simulink model "otter_traj_test"  (R2024a)
settings: Solver=FixedStepAuto  StartTime=0.0  StopTime=10.0  FixedStep=0.05  RelTol=1e-3
PostLoadFcn:
  | on_model_load
StartFcn:
  | on_model_start
StopFcn:
  | on_simulation_done
undefined symbols (not defined in the file or in its folder): ActiveScenario
libraries: csbenchlab_dist x4, mss_wrappers x3, csbenchlab_Controllers x2, ctl x1, csbenchlab_est x1, SignalEditorBlockLib x1
PostSaveFcn:
  | on_model_save
settings Model: Creator=luka  LastModifiedBy=luka

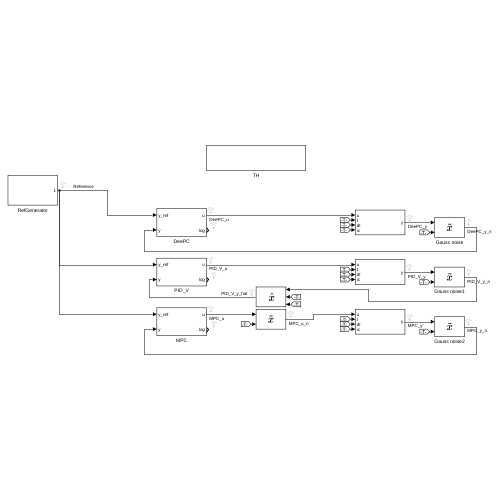
[thumbnail: Simulink's stored preview of the top-level diagram]
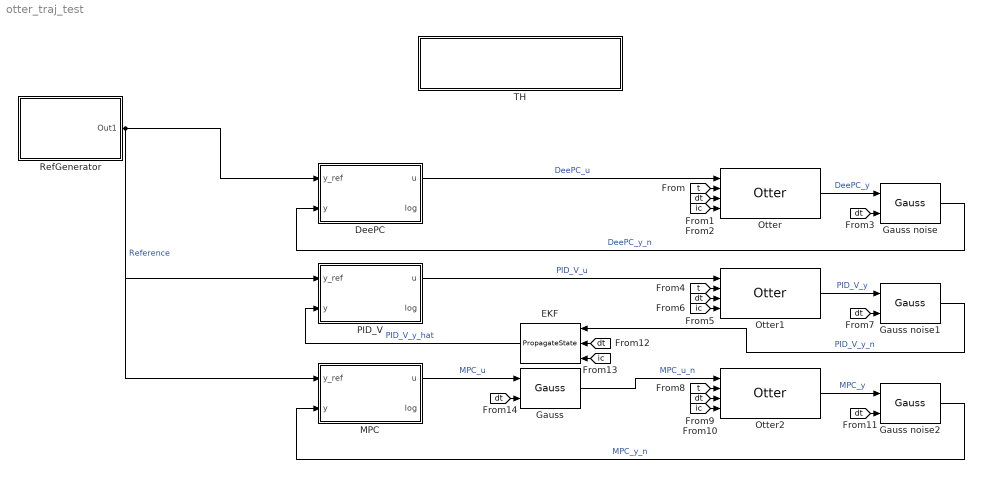
== system otter_traj_test ==
  DeePC : Subsystem
  EKF : csbenchlab_est/PropagateState  Tag=__cs_m_est;  params=PropagateState_params  data=PropagateState_data  ParamsType=PropagateState_PT  DataType=PropagateState_DT  iid__=[0]  pid__=[80 114 111 112 97 103 97 116 101 83 116 97 116 101 58 99 115 98 101 110 99 104 108 97 98]
  Gauss : csbenchlab_dist/Gauss  Tag=__cs_m_dist;  params=Gauss_params  data=Gauss_data  ParamsType=Gauss_PT  DataType=Gauss_DT  iid__=[0]  pid__=[71 97 117 115 115 58 99 115 98 101 110 99 104 108 97 98]
  Gauss noise : csbenchlab_dist/Gauss  Tag=__cs_m_dist;  params=Gauss_params  data=Gauss_data  ParamsType=Gauss_PT  DataType=Gauss_DT  iid__=[0]  pid__=[71 97 117 115 115 58 99 115 98 101 110 99 104 108 97 98]
  Gauss noise1 : csbenchlab_dist/Gauss  Tag=__cs_m_dist;  params=Gauss_params  data=Gauss_data  ParamsType=Gauss_PT  DataType=Gauss_DT  iid__=[0]  pid__=[71 97 117 115 115 58 99 115 98 101 110 99 104 108 97 98]
  Gauss noise2 : csbenchlab_dist/Gauss  Tag=__cs_m_dist;  params=Gauss_params  data=Gauss_data  ParamsType=Gauss_PT  DataType=Gauss_DT  iid__=[0]  pid__=[71 97 117 115 115 58 99 115 98 101 110 99 104 108 97 98]
  MPC : Subsystem
  Otter : mss_wrappers/Otter  Tag=system;__cs_slx_sys;  params=Otter_params_bkp  merged_params=ActiveScenario.Params
  Otter1 : mss_wrappers/Otter  Tag=system;__cs_slx_sys;  params=Otter_params_bkp  merged_params=ActiveScenario.Params
  Otter2 : mss_wrappers/Otter  Tag=system;__cs_slx_sys;  params=Otter_params_bkp  merged_params=ActiveScenario.Params
  PID_V : Subsystem
  RefGenerator : Subsystem  mask{scenario=P1}
      settings: OpenFcn=on_reference_generator_open();
      mask TypeOptions scenario: P1
      mask Callback scenario: on_reference_select;
      mask DialogControl edit_refs_btn Prompt: Edit references
      mask DialogControl edit_refs_btn Callback: on_edit_references_btn;
  TH : Subsystem
      mask DialogControl ParameterGroupVar Prompt: Params
  wires:
  [t] -> Otter/2
  [dt] -> Otter/3
  [ic] -> Otter/4
  [dt] -> Gauss noise/2
  [t] -> Otter1/2
  [dt] -> Otter1/3
  [ic] -> Otter1/4
  [dt] -> Gauss noise1/2
  [t] -> Otter2/2
  [dt] -> Otter2/3
  [ic] -> Otter2/4
  [dt] -> Gauss noise2/2
  [dt] -> EKF/2
  [ic] -> EKF/3
  [dt] -> Gauss/2
  DeePC/1(u) -> Otter/1  "DeePC_u"
  Otter/1 -> Gauss noise/1  "DeePC_y"
  Gauss noise/1 -> DeePC/2(y)  "DeePC_y_n"
  RefGenerator/1(Out1) -> DeePC/1(y_ref), PID_V/1(y_ref), MPC/1(y_ref)  "Reference"
  PID_V/1(u) -> Otter1/1  "PID_V_u"
  Otter1/1 -> Gauss noise1/1  "PID_V_y"
  Gauss noise1/1 -> EKF/1  "PID_V_y_n"
  EKF/1 -> PID_V/2(y)  "PID_V_y_hat"
  MPC/1(u) -> Gauss/1  "MPC_u"
  Gauss/1 -> Otter2/1  "MPC_u_n"
  Otter2/1 -> Gauss noise2/1  "MPC_y"
  Gauss noise2/1 -> MPC/2(y)  "MPC_y_n"

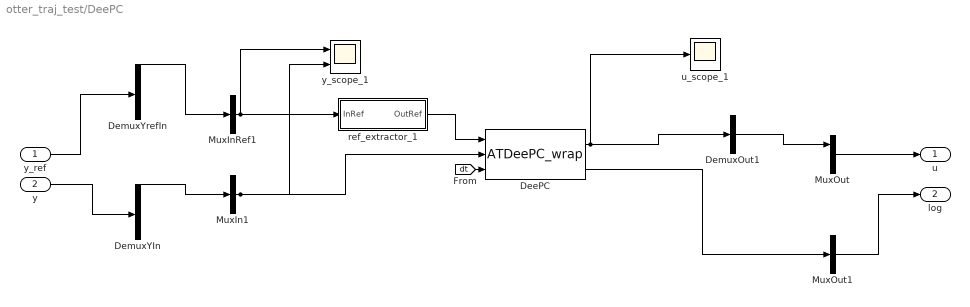
== system otter_traj_test/DeePC ==
  y_ref : Inport  PortDimensions=12
  y : Inport  Port=2  PortDimensions=12
  DeePC : ctl/ATDeePC_wrap  Tag=controller;__cs_slx_ctl;  params=ATDeePC_params  trajectory_T=0  data=0  db_params=0
  DemuxOut1 : Demux  Outputs=1
  DemuxYIn : Demux  Outputs=12
  DemuxYrefIn : Demux  Outputs=12
  MuxIn1 : Mux  Inputs=1
  MuxInRef1 : Mux  Inputs=1
  MuxOut : Mux  Inputs=2
  MuxOut1 : BusCreator  Inputs=1
  ref_extractor_1 : Subsystem
  u_scope_1 : Scope
  y_scope_1 : Scope  NumInputPorts=2
  u : Outport  PortDimensions=2
  log : Outport  Port=2
  wires:
  [dt] -> DeePC/3
  y/1 -> DemuxYIn/1
  y_ref/1 -> DemuxYrefIn/1
  MuxOut/1 -> u/1
  MuxOut1/1 -> log/1
  MuxInRef1/1 -> ref_extractor_1/1(InRef), y_scope_1/1
  ref_extractor_1/1(OutRef) -> DeePC/1
  MuxIn1/1 -> DeePC/2, y_scope_1/2
  DeePC/1 -> DemuxOut1/1, u_scope_1/1
  DeePC/2 -> MuxOut1/1
  DemuxYIn/1 -> MuxIn1/1
  DemuxYrefIn/1 -> MuxInRef1/1
  DemuxOut1/1 -> MuxOut/1

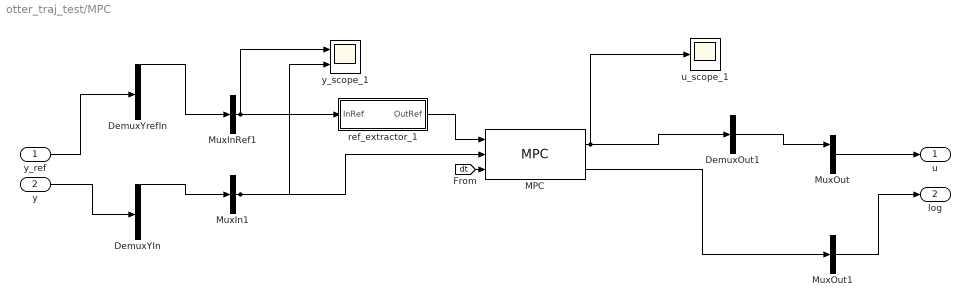
== system otter_traj_test/MPC ==
  y_ref : Inport  PortDimensions=12
  y : Inport  Port=2  PortDimensions=12
  DemuxOut1 : Demux  Outputs=1
  DemuxYIn : Demux  Outputs=12
  DemuxYrefIn : Demux  Outputs=12
  MPC : csbenchlab_Controllers/MPC  Tag=__cs_slx_ctl;  params=MPC_params
  MuxIn1 : Mux  Inputs=1
  MuxInRef1 : Mux  Inputs=1
  MuxOut : Mux  Inputs=2
  MuxOut1 : BusCreator  Inputs=1
  ref_extractor_1 : Subsystem
  u_scope_1 : Scope
  y_scope_1 : Scope  NumInputPorts=2
  u : Outport  PortDimensions=2
  log : Outport  Port=2
  wires:
  [dt] -> MPC/3
  y/1 -> DemuxYIn/1
  y_ref/1 -> DemuxYrefIn/1
  MuxOut/1 -> u/1
  MuxOut1/1 -> log/1
  MuxInRef1/1 -> ref_extractor_1/1(InRef), y_scope_1/1
  ref_extractor_1/1(OutRef) -> MPC/1
  MuxIn1/1 -> MPC/2, y_scope_1/2
  MPC/1 -> DemuxOut1/1, u_scope_1/1
  MPC/2 -> MuxOut1/1
  DemuxYIn/1 -> MuxIn1/1
  DemuxYrefIn/1 -> MuxInRef1/1
  DemuxOut1/1 -> MuxOut/1

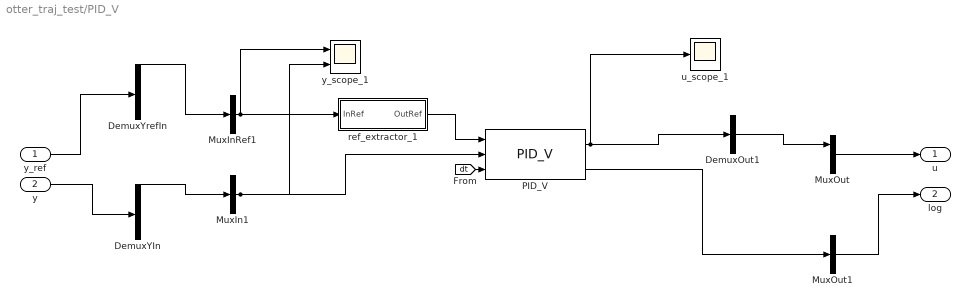
== system otter_traj_test/PID_V ==
  y_ref : Inport  PortDimensions=12
  y : Inport  Port=2  PortDimensions=12
  DemuxOut1 : Demux  Outputs=1
  DemuxYIn : Demux  Outputs=12
  DemuxYrefIn : Demux  Outputs=12
  MuxIn1 : Mux  Inputs=1
  MuxInRef1 : Mux  Inputs=1
  MuxOut : Mux  Inputs=2
  MuxOut1 : BusCreator  Inputs=1
  PID_V : csbenchlab_Controllers/PID_V  Tag=__cs_slx_ctl;  params=pid_params_v
  ref_extractor_1 : Subsystem
  u_scope_1 : Scope
  y_scope_1 : Scope  NumInputPorts=2
  u : Outport  PortDimensions=2
  log : Outport  Port=2
  wires:
  [dt] -> PID_V/3
  y/1 -> DemuxYIn/1
  y_ref/1 -> DemuxYrefIn/1
  MuxOut/1 -> u/1
  MuxOut1/1 -> log/1
  MuxInRef1/1 -> ref_extractor_1/1(InRef), y_scope_1/1
  ref_extractor_1/1(OutRef) -> PID_V/1
  MuxIn1/1 -> PID_V/2, y_scope_1/2
  PID_V/1 -> DemuxOut1/1, u_scope_1/1
  PID_V/2 -> MuxOut1/1
  DemuxYIn/1 -> MuxIn1/1
  DemuxYrefIn/1 -> MuxInRef1/1
  DemuxOut1/1 -> MuxOut/1

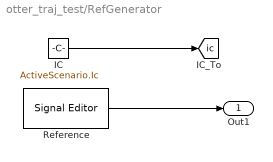
== system otter_traj_test/RefGenerator ==
  IC : Constant  Value=ActiveScenario.Ic
  Reference : SignalEditorBlockLib/Signal Editor  FileName=untitled.mat  ActiveScenario=Scenario  ActiveSignal=Signal 1  IsBus=off  OutputBusObjectStr=Bus: BusObject  SampleTime=0  Interpolate=off  ZeroCross=off  OutputAfterFinalValue=Setting to zero  Unit=inherit  PreserveSignalName=on  ApplySigPropsToAllScenarios=on  ApplySigPropsToAllSignals=off
  Out1 : Outport
  tag scope: ic=global
  wires:
  IC/1 -> [ic]
  Reference/1 -> Out1/1

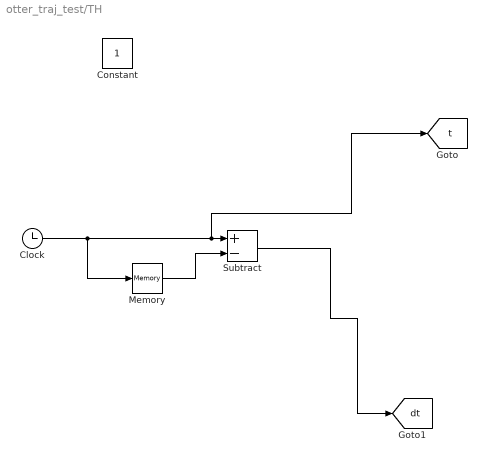
== system otter_traj_test/TH ==
  Clock : Clock
  Constant : Constant
  Memory : Memory
  Subtract : Sum  Inputs=+-
  tag scope: dt=global, t=global
  wires:
  Subtract/1 -> [dt]
  Memory/1 -> Subtract/2
  Clock/1 -> Memory/1, Subtract/1, [t]

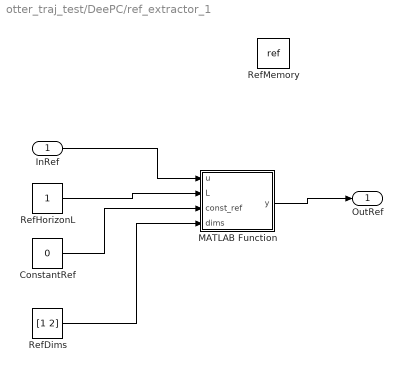
== system otter_traj_test/DeePC/ref_extractor_1 ==
  InRef : Inport
  ConstantRef : Constant  Value=0
  MATLAB Function : MATLAB Function  TreatAsAtomicUnit=on
  RefDims : Constant  Value=[1 2]
  RefHorizonL : Constant
  RefMemory : DataStoreMemory  DataStoreName=ref  WriteAfterWriteMsg=warning  ShowAdditionalParam=off  OutDataTypeStr=double
  OutRef : Outport
  wires:
  ConstantRef/1 -> MATLAB Function/3(const_ref)
  RefDims/1 -> MATLAB Function/4(dims)
  RefHorizonL/1 -> MATLAB Function/2(L)
  InRef/1 -> MATLAB Function/1(u)
  MATLAB Function/1(y) -> OutRef/1

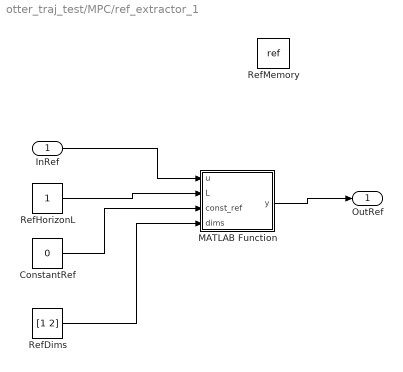
== system otter_traj_test/MPC/ref_extractor_1 ==
  InRef : Inport
  ConstantRef : Constant  Value=0
  MATLAB Function : MATLAB Function  TreatAsAtomicUnit=on
  RefDims : Constant  Value=[1 2]
  RefHorizonL : Constant
  RefMemory : DataStoreMemory  DataStoreName=ref  WriteAfterWriteMsg=warning  ShowAdditionalParam=off  OutDataTypeStr=double
  OutRef : Outport
  wires:
  ConstantRef/1 -> MATLAB Function/3(const_ref)
  RefDims/1 -> MATLAB Function/4(dims)
  RefHorizonL/1 -> MATLAB Function/2(L)
  InRef/1 -> MATLAB Function/1(u)
  MATLAB Function/1(y) -> OutRef/1

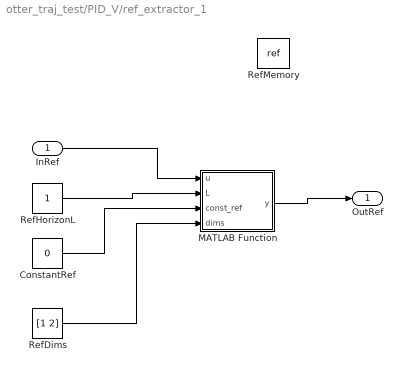
== system otter_traj_test/PID_V/ref_extractor_1 ==
  InRef : Inport
  ConstantRef : Constant  Value=0
  MATLAB Function : MATLAB Function  TreatAsAtomicUnit=on
  RefDims : Constant  Value=[1 2]
  RefHorizonL : Constant
  RefMemory : DataStoreMemory  DataStoreName=ref  WriteAfterWriteMsg=warning  ShowAdditionalParam=off  OutDataTypeStr=double
  OutRef : Outport
  wires:
  ConstantRef/1 -> MATLAB Function/3(const_ref)
  RefDims/1 -> MATLAB Function/4(dims)
  RefHorizonL/1 -> MATLAB Function/2(L)
  InRef/1 -> MATLAB Function/1(u)
  MATLAB Function/1(y) -> OutRef/1

== matlab function otter_traj_test/PID_V/ref_extractor_1/MATLAB Function ==
  settings: updateMethod=DISCRETE
  data: u input; L input; const_ref input; dims input; y output; ref data_store_memory; GlobalReference parameter
function y = fcn(u, L, const_ref, dims, GlobalReference)

persistent cnt
global ref

if isempty(cnt)
    cnt = 0;
end
cnt = cnt+1;

horizon_end = cnt+L-1;
if L > 1 
   if horizon_end > length(GlobalReference)
        if size(ref, 1) == size(u, 1)
            y = permute(ref, [2, 1]);
        else
            y = ref;
        end       
        return
   end

   if size(ref, 1) == size(u, 1)
      
      if const_ref == 0
        ref(:, :) = GlobalReference(cnt:horizon_end, dims)';
      else
        ref(:, :) = repmat(GlobalReference(cnt, dims)', 1, L);
      end
      y = permute(ref, [2, 1]);
   else
      if const_ref == 0
        ref(1:L, :) = GlobalReference(cnt:horizon_end, dims);
      else
        ref(1:L, :) = repmat(GlobalReference(cnt, dims), L, 1);
      end
      y = ref;
   end
else
   if size(ref, 1) == size(u, 1)
       ref = u;
       y = permute(ref, [2, 1]);
   else
      ref(1, :) = u';
      y = ref;
   end
end

== matlab function otter_traj_test/MPC/ref_extractor_1/MATLAB Function ==
  settings: updateMethod=DISCRETE
  data: u input; L input; const_ref input; dims input; y output; ref data_store_memory; GlobalReference parameter
function y = fcn(u, L, const_ref, dims, GlobalReference)

persistent cnt
global ref

if isempty(cnt)
    cnt = 0;
end
cnt = cnt+1;

horizon_end = cnt+L-1;
if L > 1 
   if horizon_end > length(GlobalReference)
        if size(ref, 1) == size(u, 1)
            y = permute(ref, [2, 1]);
        else
            y = ref;
        end       
        return
   end

   if size(ref, 1) == size(u, 1)
      
      if const_ref == 0
        ref(:, :) = GlobalReference(cnt:horizon_end, dims)';
      else
        ref(:, :) = repmat(GlobalReference(cnt, dims)', 1, L);
      end
      y = permute(ref, [2, 1]);
   else
      if const_ref == 0
        ref(1:L, :) = GlobalReference(cnt:horizon_end, dims);
      else
        ref(1:L, :) = repmat(GlobalReference(cnt, dims), L, 1);
      end
      y = ref;
   end
else
   if size(ref, 1) == size(u, 1)
       ref = u;
       y = permute(ref, [2, 1]);
   else
      ref(1, :) = u';
      y = ref;
   end
end

== matlab function otter_traj_test/DeePC/ref_extractor_1/MATLAB Function ==
  settings: updateMethod=DISCRETE
  data: u input; L input; const_ref input; dims input; y output; ref data_store_memory; GlobalReference parameter
function y = fcn(u, L, const_ref, dims, GlobalReference)

persistent cnt
global ref

if isempty(cnt)
    cnt = 0;
end
cnt = cnt+1;

horizon_end = cnt+L-1;
if L > 1 
   if horizon_end > length(GlobalReference)
        if size(ref, 1) == size(u, 1)
            y = permute(ref, [2, 1]);
        else
            y = ref;
        end       
        return
   end

   if size(ref, 1) == size(u, 1)
      
      if const_ref == 0
        ref(:, :) = GlobalReference(cnt:horizon_end, dims)';
      else
        ref(:, :) = repmat(GlobalReference(cnt, dims)', 1, L);
      end
      y = permute(ref, [2, 1]);
   else
      if const_ref == 0
        ref(1:L, :) = GlobalReference(cnt:horizon_end, dims);
      else
        ref(1:L, :) = repmat(GlobalReference(cnt, dims), L, 1);
      end
      y = ref;
   end
else
   if size(ref, 1) == size(u, 1)
       ref = u;
       y = permute(ref, [2, 1]);
   else
      ref(1, :) = u';
      y = ref;
   end
end
